simulink model "Microgrid_ITM_server"  (R2025b)
settings: Solver=FixedStepAuto  StartTime=0.0  StopTime=0.05  FixedStep=5e-7  RelTol=1e-3
InitFcn:
  | clear;
  | setup_two_pc_cosim();
  | clear Server_co Client_co
  | rehash;
  | release_two_pc_tcp_ports();
  | Vline = 380;%Rated RMS of Line Voltage
  | Vdc = 750;%DC voltage
  | Vac = sqrt(2)*Vline/sqrt(3);%Amplitude of Phase to Neutral Volatge
  | P = 10*10^(3);%Rate Power
  | f=50;%Rated Frequency
  | Wb=2*pi*f;%Rated Angular Frequency
  | fsw1=10e3;  %INV1 switching frequency
  | 
  | %Base Value of PU System
  | Vp=Vac;%Voltage
  | Ip=2/3*P/Vp;%Current
  | Zb = Vp/Ip;%Impedance
  | Lb=Zb/2/pi/f;%Inductance
  | Cb=1/(2*pi*f*Zb);%Capacitance
  | 
  | %Network Parameters
  | R1_pu=0.1/Zb;R1=R1_pu*Zb;
  | R2_pu=0.1/Zb;R2=R2_pu*Zb;
  | R3_pu=0.1/Zb;R3=R3_pu*Zb;
  | R4_pu=0.1/Zb;R4=R4_pu*Zb;
  | L1_pu=2e-3/Lb;L1=L1_pu*Lb;
  | L2_pu=2e-3/Lb;L2=L2_pu*Lb;
  | L3_pu=2e-3/Lb;L3=L3_pu*Lb;
  | L4_pu=2e-3/Lb;L4=L4_pu*Lb;
  | 
  | %Load Parameters
  | Rload1_pu=Vp/Ip/Zb;Rload1=Rload1_pu*Zb;
  | Rload2_pu=Vp/Ip/Zb;Rload2=Rload2_pu*Zb;
  | Rload3_pu=Vp/Ip/Zb;Rload3=Rload3_pu*Zb;
  | 
  | %Virtual Impedance
  | Rv_pu=0.05;
  | Xv_pu=0.2;
  | 
  | Lc=2.5e-3;
StopFcn:
  | %% StopFcn: save ITM server-side results
  | 
  | modelName = bdroot;
  | modelFile = get_param(modelName, 'FileName');
  | 
  | if isempty(modelFile)
  |     modelDir = pwd;
  | else
  |     modelDir = fileparts(modelFile);
  | end
  | 
  | % 创建 result 文件夹
  | resultDir = fullfile(modelDir, 'result');
  | 
  | if ~exist(resultDir, 'dir')
  |     mkdir(resultDir);
  | end
  | 
  | % ITM接口服务器侧的工作区变量
  | variableNames = {
  |     'server_voltage'
  |     'server_current'
  |     'server_PQ'
  | };
  | 
  | % 添加 _server_ITM 后缀
  | ITMData = struct();
  | 
  | for k = 1:numel(variableNames)
  | 
  |     originalName = variableNames{k};
  |     saveName = [originalName, '_server_ITM'];
  | 
  |     variableExists = evalin( ...
  |         'base', ...
  |         sprintf('exist(''%s'', ''var'')', originalName));
  | 
  |     if variableExists
  |         ITMData.(saveName) = evalin('base', originalName);
  |     else
  |         warning( ...
  |             'StopFcn:MissingVariable', ...
  |             'Variable "%s" was not found in the base workspace.', ...
  |             originalName);
  |     end
  | end
  | 
  | % 保存到 result/server_ITM.mat
  | saveFile = fullfile(resultDir, 'server_ITM.mat');
  | save(saveFile, '-struct', 'ITMData');
  | 
  | fprintf('ITM server-side results saved to:\n%s\n', saveFile);
undefined symbols (not defined in the file or in its folder): DiscIntNeverNeededParam, Lline1
libraries: spsThreePhaseSeriesRLCBranchLib x13, spsControlledVoltageSourceLib x12, spsThreePhaseVIMeasurementLib x7, spsControlledCurrentSourceLib x6, spsabctodq0Lib x6, slpidlib x4, spsThreePhaseBreakerLib x4, SimplusGT x3, spsPower3phInstantaneousLib x2, spsdq0toabcLib x2, spsThreePhaseTransformerTwoWindingsLib x2, spsDistributedParametersLineLib x1
(part 2 of 2)

== system Microgrid_ITM_server/Subsystem/LOAD4 ==
  Constant1 : Constant
  Rload2 : spsThreePhaseSeriesRLCBranchLib/Three-Phase Series RLC Branch  LConnTagsString=A|B|C  RConnTagsString=A|B|C  BranchType=R  Resistance=Rload2  Inductance=Lline1  Capacitance=1e-6  Measurements=None
  Three-Phase Breaker1 : spsThreePhaseBreakerLib/Three-Phase Breaker  InitialState=open  SwitchA=on  SwitchB=on  SwitchC=on  SwitchTimes=1.5  External=on  BreakerResistance=0.01  SnubberResistance=1e6  SnubberCapacitance=inf  Measurements=None
  A : PMIOPort  Side=Left
  B : PMIOPort  Port=2  Side=Left
  C : PMIOPort  Port=3  Side=Left
  wires:
  Constant1/1 -> Three-Phase Breaker1/1
  connections:
  Three-Phase Breaker1/RConn3 -- Rload2/LConn3
  B/RConn1 -- Three-Phase Breaker1/LConn2
  Three-Phase Breaker1/RConn1 -- Rload2/LConn1
  C/RConn1 -- Three-Phase Breaker1/LConn3
  Rload2/RConn3 -- Rload2/RConn2 -- Rload2/RConn1
  Three-Phase Breaker1/RConn2 -- Rload2/LConn2
  A/RConn1 -- Three-Phase Breaker1/LConn1

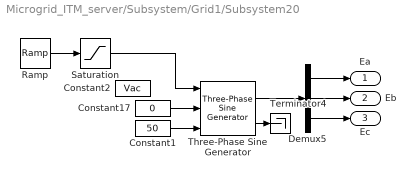
== system Microgrid_ITM_server/Subsystem/Grid1/Subsystem20 ==
  Constant1 : Constant  Value=50
  Constant17 : Constant  Value=0
  Constant2 : Constant  Value=Vac
  Demux5 : Demux  Outputs=3
  Ramp : simulink/Sources/Ramp  slope=Vac/0.01  start=0  InitialOutput=0
  Saturation : Saturate  UpperLimit=Vac  LowerLimit=0
  Terminator4 : Terminator
  Three-Phase Sine Generator : spsThreePhaseSineGeneratorLib/Three-Phase Sine Generator  Ts=1e-6
      settings: LibrarySourceBlock=|
      | sps_lib/Sources/Signal Generator Sources/Three-Phase
      | Sine Generator
  Ea : Outport
  Eb : Outport  Port=2
  Ec : Outport  Port=3
  wires:
  Three-Phase Sine Generator/1 -> Demux5/1
  Three-Phase Sine Generator/2 -> Terminator4/1
  Demux5/1 -> Ea/1
  Demux5/2 -> Eb/1
  Demux5/3 -> Ec/1
  Constant17/1 -> Three-Phase Sine Generator/2
  Constant1/1 -> Three-Phase Sine Generator/3
  Ramp/1 -> Saturation/1
  Saturation/1 -> Three-Phase Sine Generator/1

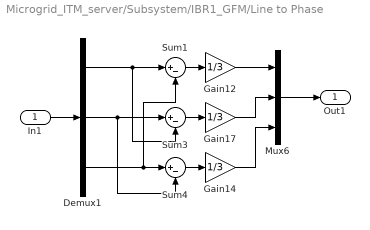
== system Microgrid_ITM_server/Subsystem/IBR1_GFM/Line to Phase ==
  In1 : Inport
  Demux1 : Demux  Outputs=3
  Gain12 : Gain  Gain=1/3
  Gain14 : Gain  Gain=1/3
  Gain17 : Gain  Gain=1/3
  Mux6 : Mux  Inputs=3
  Sum1 : Sum  Inputs=|+-
  Sum3 : Sum  Inputs=|+-
  Sum4 : Sum  Inputs=|+-
  Out1 : Outport
  wires:
  Sum3/1 -> Gain17/1
  Gain17/1 -> Mux6/2
  In1/1 -> Demux1/1
  Gain14/1 -> Mux6/3
  Sum1/1 -> Gain12/1
  Sum4/1 -> Gain14/1
  Demux1/3 -> Sum4/1, Sum1/2
  Demux1/2 -> Sum4/2, Sum3/1
  Gain12/1 -> Mux6/1
  Mux6/1 -> Out1/1
  Demux1/1 -> Sum3/2, Sum1/1

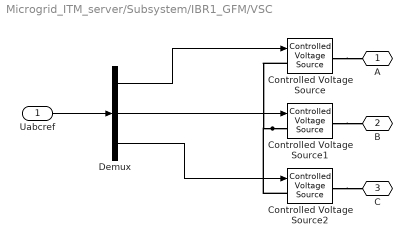
== system Microgrid_ITM_server/Subsystem/IBR1_GFM/VSC ==
  Uabcref : Inport
  Controlled Voltage Source : spsControlledVoltageSourceLib/Controlled Voltage Source  Initialize=on  Source_Type=AC  Amplitude=0  Phase=0  Frequency=0  Measurements=None
  Controlled Voltage Source1 : spsControlledVoltageSourceLib/Controlled Voltage Source  Initialize=on  Source_Type=AC  Amplitude=0  Phase=0  Frequency=0  Measurements=None
  Controlled Voltage Source2 : spsControlledVoltageSourceLib/Controlled Voltage Source  Initialize=on  Source_Type=AC  Amplitude=0  Phase=0  Frequency=0  Measurements=None
  Demux : Demux  Outputs=3
  A : PMIOPort  Side=Right
  B : PMIOPort  Port=2  Side=Right
  C : PMIOPort  Port=3  Side=Right
  wires:
  Demux/2 -> Controlled Voltage Source1/1
  Uabcref/1 -> Demux/1
  Demux/1 -> Controlled Voltage Source/1
  Demux/3 -> Controlled Voltage Source2/1
  connections:
  Controlled Voltage Source2/RConn1 -- C/RConn1
  Controlled Voltage Source1/LConn1 -- Controlled Voltage Source2/LConn1 -- Controlled Voltage Source/LConn1
  Controlled Voltage Source1/RConn1 -- B/RConn1
  Controlled Voltage Source/RConn1 -- A/RConn1

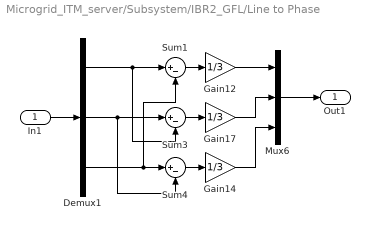
== system Microgrid_ITM_server/Subsystem/IBR2_GFL/Line to Phase ==
  In1 : Inport
  Demux1 : Demux  Outputs=3
  Gain12 : Gain  Gain=1/3
  Gain14 : Gain  Gain=1/3
  Gain17 : Gain  Gain=1/3
  Mux6 : Mux  Inputs=3
  Sum1 : Sum  Inputs=|+-
  Sum3 : Sum  Inputs=|+-
  Sum4 : Sum  Inputs=|+-
  Out1 : Outport
  wires:
  Sum3/1 -> Gain17/1
  Gain17/1 -> Mux6/2
  In1/1 -> Demux1/1
  Gain14/1 -> Mux6/3
  Sum1/1 -> Gain12/1
  Sum4/1 -> Gain14/1
  Demux1/3 -> Sum4/1, Sum1/2
  Demux1/2 -> Sum4/2, Sum3/1
  Gain12/1 -> Mux6/1
  Mux6/1 -> Out1/1
  Demux1/1 -> Sum3/2, Sum1/1

== system Microgrid_ITM_server/Subsystem/IBR2_GFL/PID ==
  In1 : Inport
  Discrete-Time Integrator : DiscreteIntegrator  gainval=5  SampleTime=-1  LimitOutput=on  UpperSaturationLimit=1.5  LowerSaturationLimit=-1.5  ICPrevOutput=DiscIntNeverNeededParam  ICPrevScaledInput=DiscIntNeverNeededParam
  Gain2 : Gain  SaturateOnIntegerOverflow=on  OutDataTypeStr=Inherit: Same as input  ParamDataTypeStr=Inherit: Same as input
  Saturation : Saturate  UpperLimit=1.5  LowerLimit=-1.5
  Sum2 : Sum  Inputs=++|
  Out1 : Outport  VectorParamsAs1DForOutWhenUnconnected=off
  wires:
  Gain2/1 -> Sum2/2
  In1/1 -> Discrete-Time Integrator/1, Gain2/1
  Sum2/1 -> Saturation/1
  Discrete-Time Integrator/1 -> Sum2/1
  Saturation/1 -> Out1/1

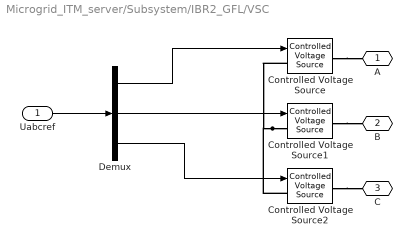
== system Microgrid_ITM_server/Subsystem/IBR2_GFL/VSC ==
  Uabcref : Inport
  Controlled Voltage Source : spsControlledVoltageSourceLib/Controlled Voltage Source  Initialize=on  Source_Type=AC  Amplitude=0  Phase=0  Frequency=0  Measurements=None
  Controlled Voltage Source1 : spsControlledVoltageSourceLib/Controlled Voltage Source  Initialize=on  Source_Type=AC  Amplitude=0  Phase=0  Frequency=0  Measurements=None
  Controlled Voltage Source2 : spsControlledVoltageSourceLib/Controlled Voltage Source  Initialize=on  Source_Type=AC  Amplitude=0  Phase=0  Frequency=0  Measurements=None
  Demux : Demux  Outputs=3
  A : PMIOPort  Side=Right
  B : PMIOPort  Port=2  Side=Right
  C : PMIOPort  Port=3  Side=Right
  wires:
  Demux/2 -> Controlled Voltage Source1/1
  Uabcref/1 -> Demux/1
  Demux/1 -> Controlled Voltage Source/1
  Demux/3 -> Controlled Voltage Source2/1
  connections:
  Controlled Voltage Source2/RConn1 -- C/RConn1
  Controlled Voltage Source1/LConn1 -- Controlled Voltage Source/LConn1 -- Controlled Voltage Source2/LConn1
  Controlled Voltage Source1/RConn1 -- B/RConn1
  Controlled Voltage Source/RConn1 -- A/RConn1
